simulink model "Command_par_retour_etat"  (R2016a)
settings: Solver=VariableStepAuto  StartTime=0.0  StopTime=20  MaxStep=0.001  RelTol=1e-3
values from neighbouring files (symbols this model uses):
  A = [0          1 0 0 ... (first row only)    [Model.m]
  B = [0 ; -1/M/L; 0; 1/M]    [Model.m]
  C = [1 0 0 0 ... (first row only)    [Model.m]
  D = [0;0]    [Model.m]
  Di = [0; 0; 0; 0]    [Model.m]
  F = acker(A,B,P)    [Model.m]
  X0 = [0.3 0 0.1 0]'    [Model.m]
undefined symbols (not defined in the file or in its folder): Ci
settings Model: Creator=NADOUR  LastModifiedBy=NADOUR

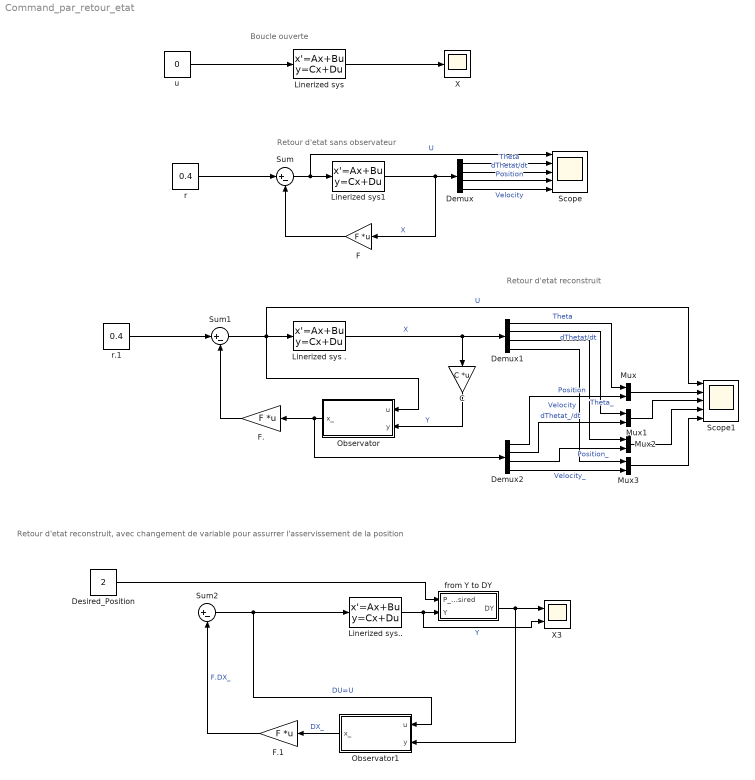
== system Command_par_retour_etat ==
  note: Retour d'etat reconstruit, avec changement de variable pour assurrer l'asservissement de la position
  note: Retour d'etat reconstruit
  note: Retour d'etat sans observateur
  note: Boucle ouverte
  C : Gain  Gain=C  Multiplication=Matrix(K*u) (u vector)
  Demux : Demux
  Demux1 : Demux
  Demux2 : Demux
  Desired_Position : Constant  Value=2
  F : Gain  Gain=F  Multiplication=Matrix(K*u) (u vector)
  F. : Gain  Gain=F  Multiplication=Matrix(K*u) (u vector)
  F.1 : Gain  Gain=F  Multiplication=Matrix(K*u) (u vector)
  Linerized sys : StateSpace  A=A  B=B  C=Ci  D=Di  X0=X0
  Linerized sys . : StateSpace  A=A  B=B  C=Ci  D=Di  X0=X0*0
  Linerized sys.. : StateSpace  A=A  B=B  C=C  D=D  X0=X0
  Linerized sys1 : StateSpace  A=A  B=B  C=Ci  D=Di  X0=X0
  Mux{,1..3} (4 alike) : Mux  Inputs=2
  Observator : Subsystem
  Observator1 : Subsystem
  Scope : Scope  NumInputPorts=5
  Scope1 : Scope  NumInputPorts=5
  Sum : Sum  Inputs=|+-
  Sum1 : Sum  Inputs=|+-
  Sum2 : Sum  Inputs=|+-
  X : Scope
  X3 : Scope  NumInputPorts=2
  from Y to DY : MATLAB Function  TreatAsAtomicUnit=on
  r : Constant  Value=0.4
  r.1 : Constant  Value=0.4
  u : Constant  Value=0
  wires:
  u/1 -> Linerized sys/1
  Linerized sys/1 -> X/1
  Sum/1 -> Scope/1, Linerized sys1/1  "U"
  Linerized sys1/1 -> Demux/1, F/1  "X"
  F/1 -> Sum/2
  Sum1/1 -> Scope1/1, Observator/1(u), Linerized sys ./1  "U"
  Linerized sys ./1 -> C/1, Demux1/1  "X"
  F./1 -> Sum1/2
  Observator/1(x_) -> F./1, Demux2/1
  Sum2/1 -> Observator1/1(u), Linerized sys../1  "DU=U"
  Linerized sys../1 -> X3/2, from Y to DY/2(Y)  "Y"
  F.1/1 -> Sum2/2  "F.DX_"
  Observator1/1(x_) -> F.1/1  "DX_"
  from Y to DY/1(DY) -> Observator1/2(y), X3/1
  Desired_Position/1 -> from Y to DY/1(P_desired)
  r/1 -> Sum/1
  r.1/1 -> Sum1/1
  Demux/1 -> Scope/2  "Theta"
  Demux/2 -> Scope/3  "dThetat/dt"
  Demux/3 -> Scope/4  "Position"
  Demux/4 -> Scope/5  "Velocity"
  C/1 -> Observator/2(y)  "Y"
  Demux1/1 -> Mux/1  "Theta"
  Demux1/2 -> Mux1/1  "dThetat/dt"
  Demux1/3 -> Mux2/1  "Position"
  Demux1/4 -> Mux3/1  "Velocity"
  Demux2/1 -> Mux/2  "Theta_"
  Demux2/2 -> Mux1/2  "dThetat_/dt"
  Demux2/3 -> Mux2/2  "Position_"
  Demux2/4 -> Mux3/2  "Velocity_"
  Mux/1 -> Scope1/2
  Mux1/1 -> Scope1/3
  Mux2/1 -> Scope1/4
  Mux3/1 -> Scope1/5

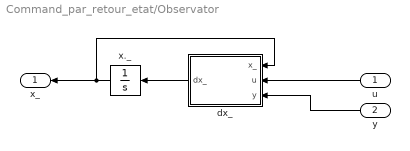
== system Command_par_retour_etat/Observator ==
  u : Inport
  y : Inport  Port=2
  dx_ : MATLAB Function  TreatAsAtomicUnit=on
  x._ : Integrator
  x_ : Outport
  wires:
  u/1 -> dx_/2(u)
  y/1 -> dx_/3(y)
  dx_/1(dx_) -> x._/1
  x._/1 -> x_/1, dx_/1(x_)

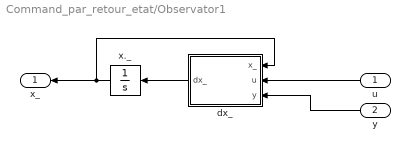
== system Command_par_retour_etat/Observator1 ==
  u : Inport
  y : Inport  Port=2
  dx_ : MATLAB Function  TreatAsAtomicUnit=on
  x._ : Integrator
  x_ : Outport
  wires:
  x._/1 -> dx_/1(x_), x_/1
  dx_/1(dx_) -> x._/1
  y/1 -> dx_/3(y)
  u/1 -> dx_/2(u)

== matlab function Command_par_retour_etat/Observator1/dx_ ==
  data: x_ input; u input; y input; dx_ output
function dx_=f(x_,u,y)
%% Parameteres:
m=0.5; M=5; L=1; g=9.8;

%% 1) The Model:
A = [0          1 0 0
    g*(m+M)/M/L 0 0 0
    0           0 0 1
    -m*g/M      0 0 0];

B = [0 ; -1/M/L; 0; 1/M];

C= [1 0 0 0
    0 0 1 0];
K =[2.9998   -0.9985
   14.7801    0.0043
    1.0015    3.0002
   -0.9757    3.9999];
%% The observation
y_=C*x_;
dx_= A*x_ + B*u + K*(y-y_);

== matlab function Command_par_retour_etat/Observator/dx_ ==
  data: x_ input; u input; y input; dx_ output
function dx_=f(x_,u,y)
%% Parameteres:
m=0.5; M=5; L=1; g=9.8;

%% 1) The Model:
A = [0          1 0 0
    g*(m+M)/M/L 0 0 0
    0           0 0 1
    -m*g/M      0 0 0];

B = [0 ; -1/M/L; 0; 1/M];

C= [1 0 0 0
    0 0 1 0];
Ks =[2.9998   -0.9985
   14.7801    0.0043
    1.0015    3.0002
   -0.9757    3.9999];
Kf =1.0e+04*[0.0300   -0.0100
            3.9992    0.0006
            0.0100    0.0300
            0.0005    4.0019];

%% The observation
y_=C*x_;
dx_= A*x_ + B*u + Ks*(y-y_);

== matlab function Command_par_retour_etat/from Y to DY ==
  data: P_desired input; DY output; Y input
function DY = fct(P_desired,Y)

DY = Y-[0; P_desired];
